simulink model "Simulink_task1"  (R2023a)
settings: Solver=VariableStepAuto  StartTime=0.0  StopTime=10.0  RelTol=1e-3
libraries: cstblocks x8
settings Model: Creator=MUHAMMAD SADEEQ  LastModifiedBy=MUHAMMAD SADEEQ

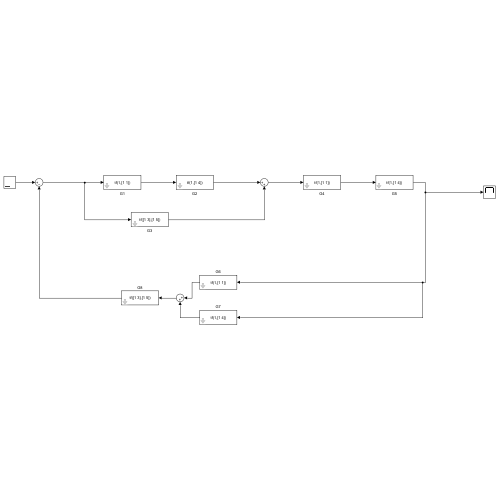
[thumbnail: Simulink's stored preview of the top-level diagram]
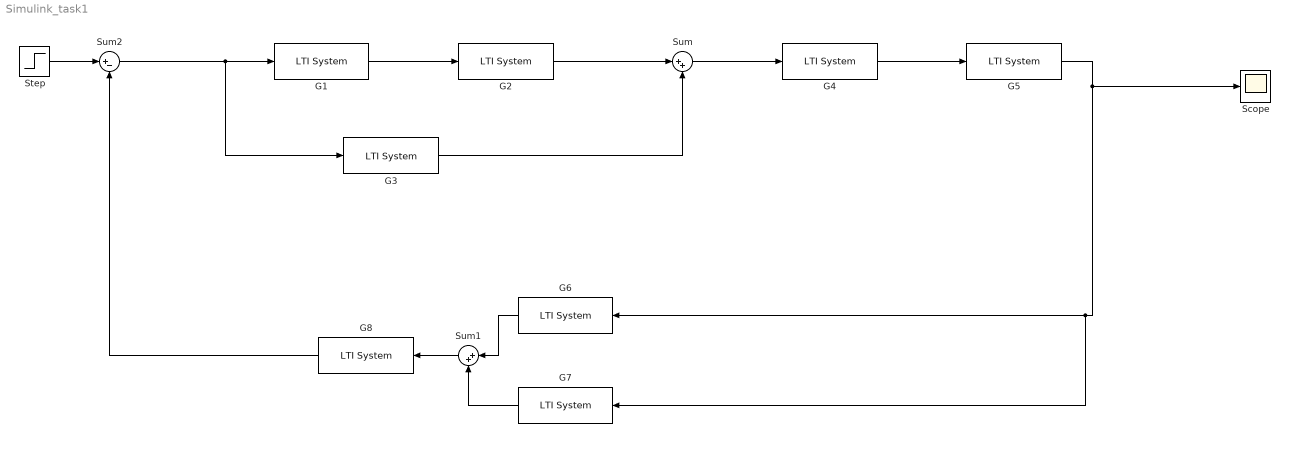
== system Simulink_task1 ==
  G1 : cstblocks/LTI System  sys=tf(1,[1 1])  IC=[]
  G2 : cstblocks/LTI System  sys=tf(1,[1 4])  IC=[]
  G3 : cstblocks/LTI System  sys=tf([1 3],[1 5])  IC=[]
  G4 : cstblocks/LTI System  sys=tf(1,[1 1])  IC=[]
  G5 : cstblocks/LTI System  sys=tf(1,[1 4])  IC=[]
  G6 : cstblocks/LTI System  sys=tf(1,[1 1])  IC=[]
  G7 : cstblocks/LTI System  sys=tf(1,[1 4])  IC=[]
  G8 : cstblocks/LTI System  sys=tf([1 3],[1 5])  IC=[]
  Scope : Scope
  Step : Step  SampleTime=0
  Sum : Sum  Inputs=|++
  Sum1 : Sum  Inputs=|++
  Sum2 : Sum  Inputs=|+-
  wires:
  G1/1 -> G2/1
  G4/1 -> G5/1
  Sum/1 -> G4/1
  G2/1 -> Sum/1
  G3/1 -> Sum/2
  G7/1 -> Sum1/2
  G6/1 -> Sum1/1
  Sum1/1 -> G8/1
  G5/1 -> Scope/1, G7/1, G6/1
  Sum2/1 -> G3/1, G1/1
  Step/1 -> Sum2/1
  G8/1 -> Sum2/2
